simulink library "gaps"  (Simulink 8.1)
settings: Solver=ode45  StartTime=0.0  StopTime=10.0  RelTol=1e-3
undefined symbols (not defined in the file or in its folder): KIFO_DefaultACCVehClearance_m, KIFO_OffsetToBumper_m, KIFO_TGapDefault_s, KIFO_TGapNoTarget_s
libraries: hcu_lib x3
settings Model: Creator=AT015126  LastModifiedBy=AT015555

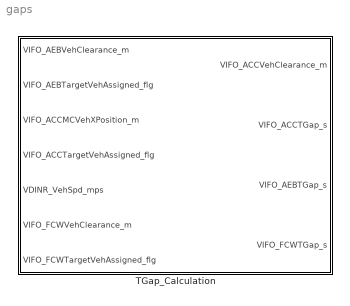
== system gaps ==
  TGap_Calculation : Subsystem

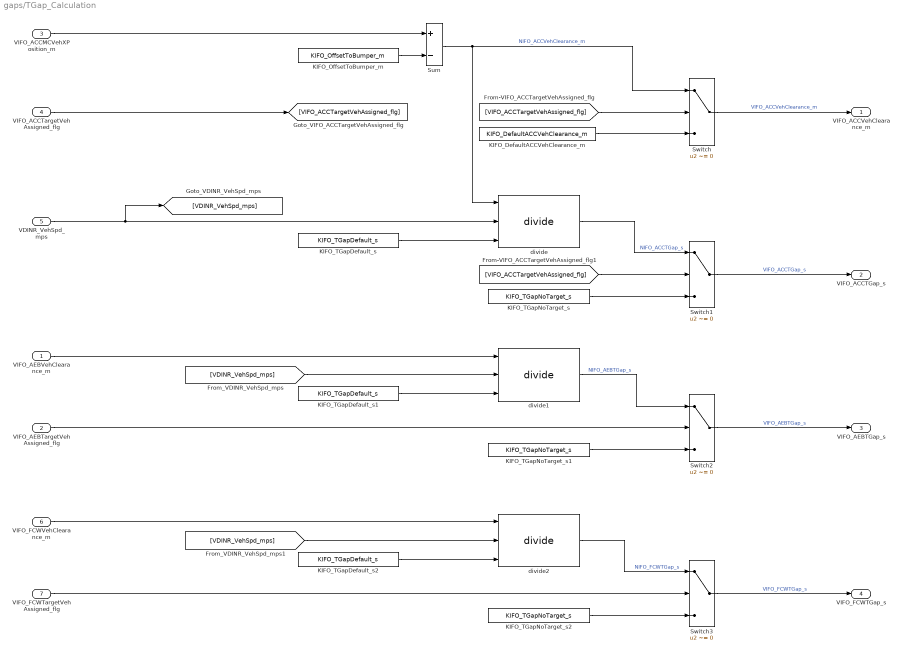
== system gaps/TGap_Calculation ==
  VIFO_AEBVehClearance_m : Inport
  VIFO_AEBTargetVehAssigned_flg : Inport  Port=2
  VIFO_ACCMCVehXPosition_m : Inport  Port=3
  VIFO_ACCTargetVehAssigned_flg : Inport  Port=4
  VDINR_VehSpd_mps : Inport  Port=5
  VIFO_FCWVehClearance_m : Inport  Port=6
  VIFO_FCWTargetVehAssigned_flg : Inport  Port=7
  KIFO_DefaultACCVehClearance_m : Constant  Value=KIFO_DefaultACCVehClearance_m
  KIFO_OffsetToBumper_m : Constant  Value=KIFO_OffsetToBumper_m
  KIFO_TGapDefault_s : Constant  Value=KIFO_TGapDefault_s
  KIFO_TGapDefault_s1 : Constant  Value=KIFO_TGapDefault_s
  KIFO_TGapDefault_s2 : Constant  Value=KIFO_TGapDefault_s
  KIFO_TGapNoTarget_s : Constant  Value=KIFO_TGapNoTarget_s
  KIFO_TGapNoTarget_s1 : Constant  Value=KIFO_TGapNoTarget_s
  KIFO_TGapNoTarget_s2 : Constant  Value=KIFO_TGapNoTarget_s
  Sum : Sum  Inputs=+-
  Switch{,1..3} (4 alike) : Switch  Criteria=u2 ~= 0
  divide : hcu_lib/divide
  divide1 : hcu_lib/divide
  divide2 : hcu_lib/divide
  VIFO_ACCVehClearance_m : Outport
  VIFO_ACCTGap_s : Outport  Port=2
  VIFO_AEBTGap_s : Outport  Port=3
  VIFO_FCWTGap_s : Outport  Port=4
  wires:
  [VDINR_VehSpd_mps] -> divide2/2
  Switch3/1 -> VIFO_FCWTGap_s/1  "VIFO_FCWTGap_s"
  KIFO_TGapDefault_s2/1 -> divide2/3
  VIFO_FCWVehClearance_m/1 -> divide2/1
  divide2/1 -> Switch3/1  "NIFO_FCWTGap_s"
  VIFO_FCWTargetVehAssigned_flg/1 -> Switch3/2
  KIFO_TGapNoTarget_s2/1 -> Switch3/3
  [VDINR_VehSpd_mps] -> divide1/2
  VDINR_VehSpd_mps/1 -> [VDINR_VehSpd_mps], divide/2
  Switch2/1 -> VIFO_AEBTGap_s/1  "VIFO_AEBTGap_s"
  KIFO_TGapDefault_s1/1 -> divide1/3
  VIFO_AEBVehClearance_m/1 -> divide1/1
  divide1/1 -> Switch2/1  "NIFO_AEBTGap_s"
  VIFO_AEBTargetVehAssigned_flg/1 -> Switch2/2
  KIFO_TGapNoTarget_s1/1 -> Switch2/3
  VIFO_ACCMCVehXPosition_m/1 -> Sum/1
  KIFO_OffsetToBumper_m/1 -> Sum/2
  Switch1/1 -> VIFO_ACCTGap_s/1  "VIFO_ACCTGap_s"
  KIFO_TGapDefault_s/1 -> divide/3
  Sum/1 -> Switch/1, divide/1  "NIFO_ACCVehClearance_m"
  VIFO_ACCTargetVehAssigned_flg/1 -> [VIFO_ACCTargetVehAssigned_flg]
  [VIFO_ACCTargetVehAssigned_flg] -> Switch/2
  KIFO_DefaultACCVehClearance_m/1 -> Switch/3
  Switch/1 -> VIFO_ACCVehClearance_m/1  "VIFO_ACCVehClearance_m"
  divide/1 -> Switch1/1  "NIFO_ACCTGap_s"
  [VIFO_ACCTargetVehAssigned_flg] -> Switch1/2
  KIFO_TGapNoTarget_s/1 -> Switch1/3
